simulink model "GCS"  (R2023a)
settings: Solver=ode1  StartTime=0.0  StopTime=inf  FixedStep=1/500  RelTol=1e-3
values from neighbouring files (symbols this model uses):
  data = uint8([                  i_int,                  i_dof,                  typecast(single(t_int), 'uint8'),                  typecast(single(coeffs), 'uint8')])    [trajectory_writer.m]    (also in ulog_plotter.m = topic.sticks(index2plot, i__).Variables)
  res = any(res)    [ulog_parser.m]
undefined symbols (not defined in the file or in its folder): f, FLIGHT_MODE, flight_mode, id, joystick, name, Parameters, timestamp, wait_time_s
libraries: simulink_extras x3, px4uORBlib x2, vrlib x1, uavmavlinklib x1, instrumentlib x1, aerolibanimutils x1
settings Model: Creator=amc0121  LastModifiedBy=yzk0058
settings DebuggingCC: UnconnectedInputMsg=warning  UnconnectedOutputMsg=warning  UnconnectedLineMsg=warning
settings ModelReferenceCC: EnableRefExpFcnMdlSchedulingChecks=on
settings RTWCC: DLArmComputeVersion=19.05

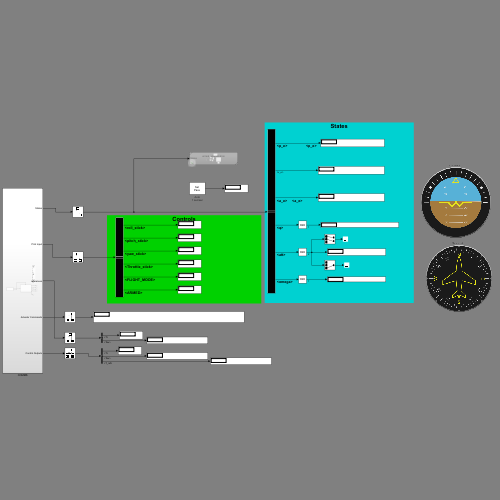
[thumbnail: Simulink's stored preview of the top-level diagram]
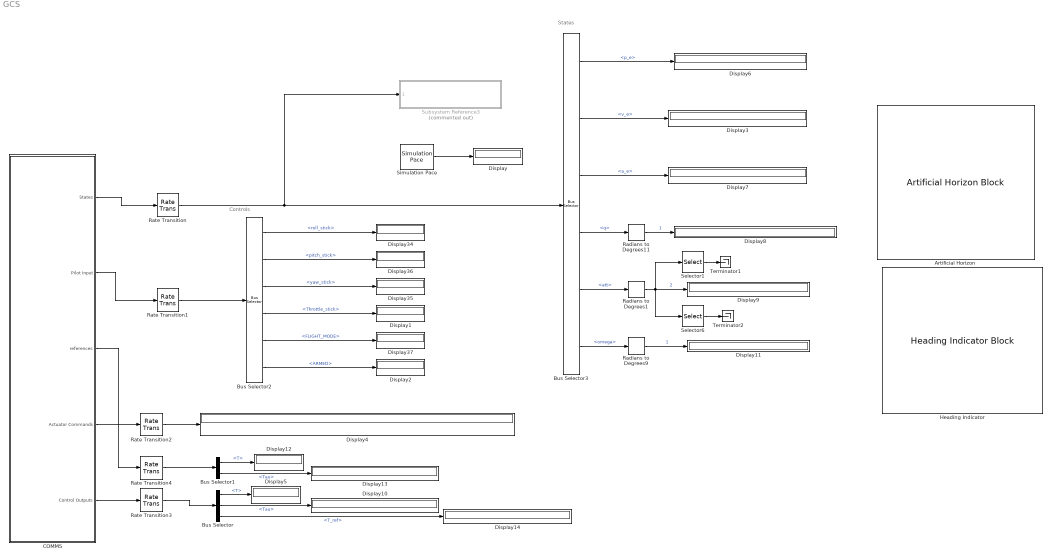
== system GCS ==
  note: Controls
  note: States
  Artificial Horizon : ArtificialHorizonBlock
  Bus Selector : BusSelector  OutputSignals=T,Tau,T_ref
  Bus Selector1 : BusSelector  OutputSignals=reconstructed.T,reconstructed.Tau
  Bus Selector2 : BusSelector  OutputSignals=Pilot Input.Sticks.roll_stick,Pilot Input.Sticks.pitch_stick,Pilot Input.Sticks.yaw_stick,Pilot Input.Sticks.Throttle_stick,Pilot Input.FLIGHT_MODE,Pilot Input.ARMED
  Bus Selector3 : BusSelector  OutputSignals=p_e,v_e,a_e,q,att,omega
  COMMS : Subsystem
  Display{,1..14,34..37} (19 alike) : Display
      Display1 settings: Decimation=30
      Display11 settings: Decimation=30
      Display2 settings: Decimation=30
      Display3 settings: Decimation=30
      Display34 settings: Decimation=30
      Display36 settings: Decimation=30
      Display37 settings: Decimation=30
      Display4 settings: Decimation=30
      Display7 settings: Decimation=30
      Display8 settings: Decimation=30
      Display9 settings: Decimation=30
  Heading Indicator : HeadingIndicatorBlock
  Radians to Degrees1 : simulink_extras/Transformations/Radians to Degrees
  Radians to Degrees11 : simulink_extras/Transformations/Radians to Degrees
  Radians to Degrees9 : simulink_extras/Transformations/Radians to Degrees
  Rate Transition{,1..4} (5 alike) : RateTransition  OutPortSampleTime=1/50
  Selector1 : Selector  InputPortWidth=3  IndexOptions=Index vector (dialog)  Indices=[1 2]  OutputSizes=1
  Selector6 : Selector  InputPortWidth=3  IndexOptions=Index vector (dialog)  Indices=[3]  OutputSizes=1
  Simulation Pace : aerolibanimutils/Simulation Pace  SimulationPace=1  SleepMode=Auto  OutputPaceError=on  SampleTime=-1
  Subsystem Reference3 : Subsystem  Commented=on  ReferencedSubsystem=unreal_visualization
  Terminator1 : Terminator
  Terminator2 : Terminator
  wires:
  Bus Selector3/1 -> Display6/1  "<p_e>"
  Bus Selector3/4 -> Radians to Degrees11/1  "<q>"
  Bus Selector3/3 -> Display7/1  "<a_e>"
  Bus Selector3/5 -> Radians to Degrees1/1  "<att>"
  Bus Selector3/6 -> Radians to Degrees9/1  "<omega>"
  Radians to Degrees9/1 -> Display11/1  "1"
  Radians to Degrees1/1 -> Selector1/1, Selector6/1, Display9/1  "2"
  Radians to Degrees11/1 -> Display8/1  "1"
  Bus Selector2/2 -> Display36/1  "<pitch_stick>"
  Bus Selector2/4 -> Display1/1  "<Throttle_stick>"
  Bus Selector2/6 -> Display2/1  "<ARMED>"
  Bus Selector2/1 -> Display34/1  "<roll_stick>"
  Bus Selector2/3 -> Display35/1  "<yaw_stick>"
  Bus Selector2/5 -> Display37/1  "<FLIGHT_MODE>"
  Simulation Pace/1 -> Display/1
  Selector1/1 -> Terminator1/1
  Selector6/1 -> Terminator2/1
  Bus Selector3/2 -> Display3/1  "<v_e>"
  COMMS/1(States) -> Rate Transition/1
  COMMS/2(Pilot Input) -> Rate Transition1/1
  COMMS/4(Actuator Commands) -> Rate Transition2/1
  Rate Transition2/1 -> Display4/1
  Rate Transition1/1 -> Bus Selector2/1
  Rate Transition/1 -> Subsystem Reference3/1, Bus Selector3/1
  COMMS/5(Control Outputs) -> Rate Transition3/1
  Rate Transition3/1 -> Bus Selector/1
  Bus Selector/1 -> Display5/1  "<T>"
  Bus Selector/2 -> Display10/1  "<Tau>"
  COMMS/3(references) -> Rate Transition4/1
  Rate Transition4/1 -> Bus Selector1/1
  Bus Selector1/1 -> Display12/1  "<T>"
  Bus Selector1/2 -> Display13/1  "<Tau>"
  Bus Selector/3 -> Display14/1  "<T_ref>"

== system GCS/COMMS ==
  note: X Input Order
      | 1. u (Vx)
      | 2. v (Vy)
      | 3. w (Vz)
      | 4. p
      | 5. q
      | 6. r
      | 7. e0
      | 8. e1
      | 9. e2
      | 10. e3
      | 11. Lat
      | 12. Long
      | 13. hMSL
      | 14. hAGL
      | 15. ax
      | 16. ay
      | 17. az
      | 18. x
      | 19. y
      | 20. z
      | 21. hdot (VV)
      | 22. GCFlag
      | 23. TAS
      | 24. EAS
      | 25. LiDAR
  Enabled Subsystem : Subsystem  TreatAsAtomicUnit=on
  UDP Receive : instrumentlib/UDP Receive  LocalAddress=127.0.0.1  LocalPort=14445  EnablePortSharing=off  Host=localhost  Port=9090  GetLatestData=off  DataSize=8  DataType=uint8  ASCIIFormatting=%f,  Terminator=LF  CustomTerminator=10  ByteOrder=big-endian  EnableBlockingMode=off  Timeout=1/300  SampleTime=1/500  SimulateUsing=Interpreted execution
  States : Outport
  Pilot Input : Outport  Port=2
  references : Outport  Port=3
  Actuator Commands : Outport  Port=4
  Control Outputs : Outport  Port=5
  wires:
  UDP Receive/2 -> Enabled Subsystem/Enable
  UDP Receive/1 -> Enabled Subsystem/1(byteStreamInput)
  Enabled Subsystem/1(States) -> States/1
  Enabled Subsystem/2(Pilot Input) -> Pilot Input/1
  Enabled Subsystem/3(references) -> references/1
  Enabled Subsystem/4(Actuator Commands) -> Actuator Commands/1
  Enabled Subsystem/5(Control Outputs) -> Control Outputs/1

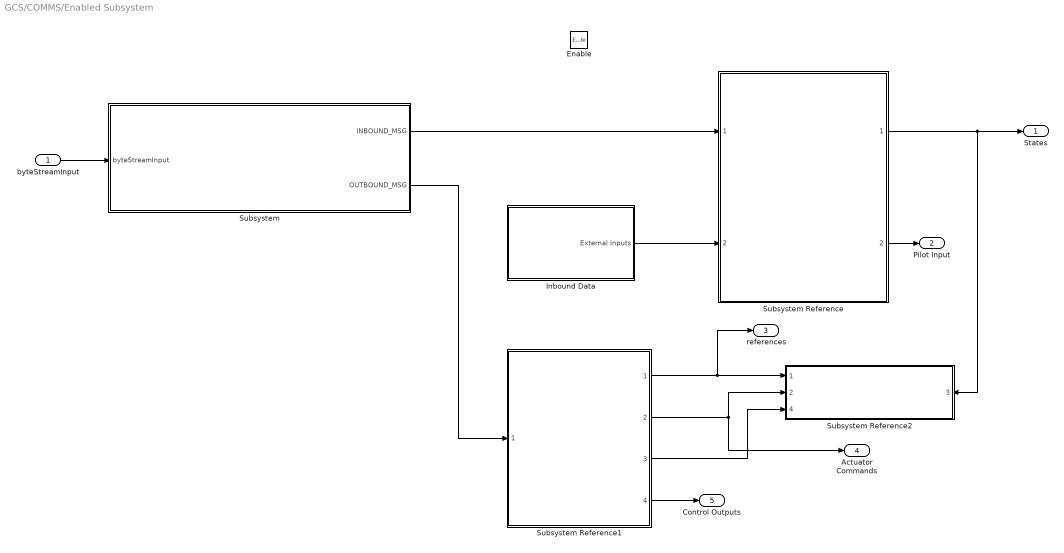
== system GCS/COMMS/Enabled Subsystem ==
  byteStreamInput : Inport
  Enable : EnablePort
  Inbound Data : Subsystem
  Subsystem : Subsystem
  Subsystem Reference : Subsystem  ReferencedSubsystem=INBOUND_MSG_UNMAP
  Subsystem Reference1 : Subsystem  ReferencedSubsystem=OUTBOUND_MSG_UNMAP
  Subsystem Reference2 : Subsystem  ReferencedSubsystem=logging2workspace
      settings: PortSchema="{\"entries\":[{\"content\":{\"sides\":[{\"content\":{\"connectorIds\":[\"In1\",\"In2\",\"In4\"]},\"type\":\"ConnectorPlacement.EquallySpacedRectSide\",\"uuid\":\"47b0435c-4974-4dfb-aae6-6ca620e26367\"},{\"content\":{\"connectorIds\":[\"In3\"],\"side\":\"RIGHT\"},\"type\":\"ConnectorPlacement.EquallySpacedRectSide\",\"uuid\":\"e323305f-4ea2-4fd9-9ec2-838e165181fb\"},{\"content\":{\"side\":\"TOP\"},\"type\":\"ConnectorPlacement.EquallySpacedRectSide\",\"uuid\":\"bec00405-cbc9-4439-89df-ad1a7655b850\"}]},\"type\":\"ConnectorPlacement.EquallySpacedConnector\",\"uuid\":\"1e7e1f21-3d1e-40b5-a907-670aed2a63f6\"}],\"packageUris\":[\"http://schema.mathworks.com/mf0/Connector/R2020b\"],\"version\":\"1.0\"}"
  States : Outport
  Pilot Input : Outport  Port=2
  references : Outport  Port=3
  Actuator Commands : Outport  Port=4
  Control Outputs : Outport  Port=5
  wires:
  byteStreamInput/1 -> Subsystem/1(byteStreamInput)
  Subsystem/2(OUTBOUND_MSG) -> Subsystem Reference1/1
  Subsystem/1(INBOUND_MSG) -> Subsystem Reference/1
  Inbound Data/1("External Inputs ") -> Subsystem Reference/2
  Subsystem Reference/1 -> States/1, Subsystem Reference2/3
  Subsystem Reference1/1 -> references/1, Subsystem Reference2/1
  Subsystem Reference/2 -> Pilot Input/1
  Subsystem Reference1/2 -> Actuator Commands/1, Subsystem Reference2/2
  Subsystem Reference1/3 -> Subsystem Reference2/4
  Subsystem Reference1/4 -> Control Outputs/1

== system GCS/COMMS/Enabled Subsystem/Inbound Data ==
  Bus Creator3 : BusCreator  Inputs=4
  Subsystem1 : Subsystem
  Subsystem2 : Subsystem
  Subsystem3 : Subsystem
  Subsystem4 : Subsystem
  "External Inputs " : Outport
  wires:
  Bus Creator3/1 -> "External Inputs "/1
  Subsystem1/1(Control Gains) -> Bus Creator3/2  "Control Gains"
  Subsystem2/1(Vehicle Parameters) -> Bus Creator3/1  "Vehicle Parameters"
  Subsystem3/1(Trajectory) -> Bus Creator3/3  "Trajectory"
  Subsystem4/1(Pilot Input) -> Bus Creator3/4  "Pilot Input"

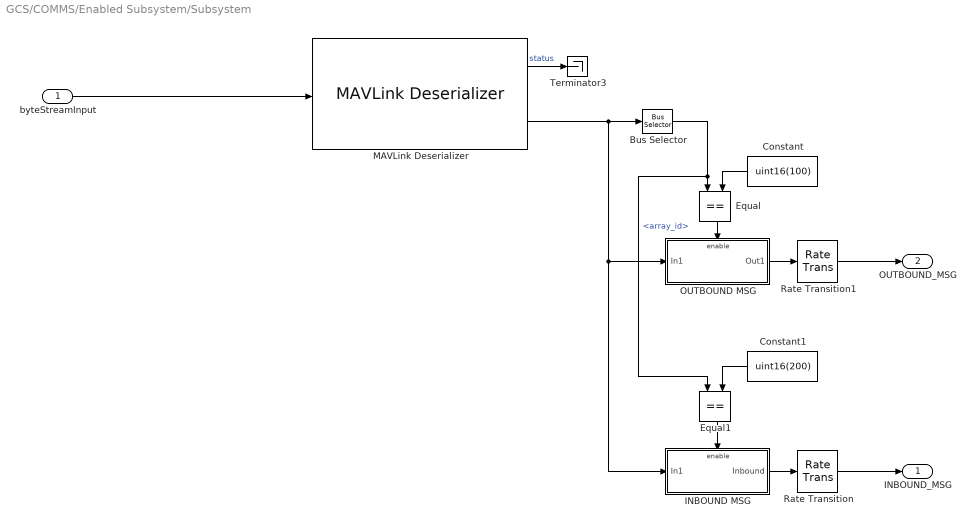
== system GCS/COMMS/Enabled Subsystem/Subsystem ==
  byteStreamInput : Inport
  Bus Selector : BusSelector  OutputSignals=Payload.array_id
  Constant : Constant  Value=uint16(100)
  Constant1 : Constant  Value=uint16(200)
  Equal : RelationalOperator  Operator===  OutDataTypeStr=boolean  RndMeth=Simplest  InputSameDT=off
  Equal1 : RelationalOperator  Operator===  OutDataTypeStr=boolean  RndMeth=Simplest  InputSameDT=off
  INBOUND MSG : Subsystem  TreatAsAtomicUnit=on
  MAVLink Deserializer : uavmavlinklib/MAVLink Deserializer  dialectSource=Select from standard MAVLink dialects  dialect=common.xml  dialectCustom=common.xml  version=2  messageType=DEBUG_FLOAT_ARRAY  inputDataLength=off  SystemIDFilter=off  systemID=1  ComponentIDFilter=off  componentID=1  queueMsg=off  queueMsgSize=50  dropNum=off
  OUTBOUND MSG : Subsystem  TreatAsAtomicUnit=on
  Rate Transition : RateTransition  OutPortSampleTime=1/25
  Rate Transition1 : RateTransition  OutPortSampleTime=1/25
  Terminator3 : Terminator
  INBOUND_MSG : Outport
  OUTBOUND_MSG : Outport  Port=2
  wires:
  Equal1/1 -> INBOUND MSG/Enable
  INBOUND MSG/1(Inbound) -> Rate Transition/1
  OUTBOUND MSG/1(Out1) -> Rate Transition1/1
  MAVLink Deserializer/2 -> INBOUND MSG/1(In1), OUTBOUND MSG/1(In1), Bus Selector/1
  Bus Selector/1 -> Equal1/1, Equal/1  "<array_id>"
  Constant/1 -> Equal/2
  Equal/1 -> OUTBOUND MSG/Enable
  Rate Transition/1 -> INBOUND_MSG/1
  MAVLink Deserializer/1 -> Terminator3/1  "status"
  Constant1/1 -> Equal1/2
  byteStreamInput/1 -> MAVLink Deserializer/1
  Rate Transition1/1 -> OUTBOUND_MSG/1

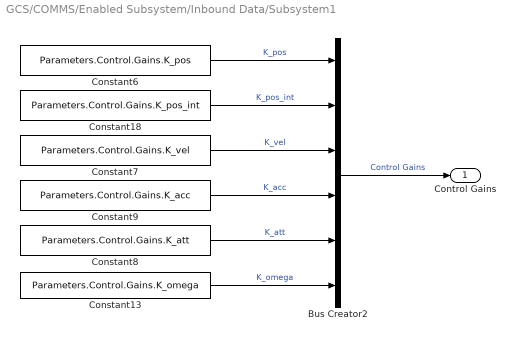
== system GCS/COMMS/Enabled Subsystem/Inbound Data/Subsystem1 ==
  Bus Creator2 : BusCreator  Inputs=6
  Constant13 : Constant  Value=Parameters.Control.Gains.K_omega
  Constant18 : Constant  Value=Parameters.Control.Gains.K_pos_int
  Constant6 : Constant  Value=Parameters.Control.Gains.K_pos
  Constant7 : Constant  Value=Parameters.Control.Gains.K_vel
  Constant8 : Constant  Value=Parameters.Control.Gains.K_att
  Constant9 : Constant  Value=Parameters.Control.Gains.K_acc
  Control Gains : Outport
  wires:
  Constant7/1 -> Bus Creator2/3  "K_vel"
  Constant6/1 -> Bus Creator2/1  "K_pos"
  Constant13/1 -> Bus Creator2/6  "K_omega"
  Bus Creator2/1 -> Control Gains/1  "Control Gains"
  Constant18/1 -> Bus Creator2/2  "K_pos_int"
  Constant9/1 -> Bus Creator2/4  "K_acc"
  Constant8/1 -> Bus Creator2/5  "K_att"

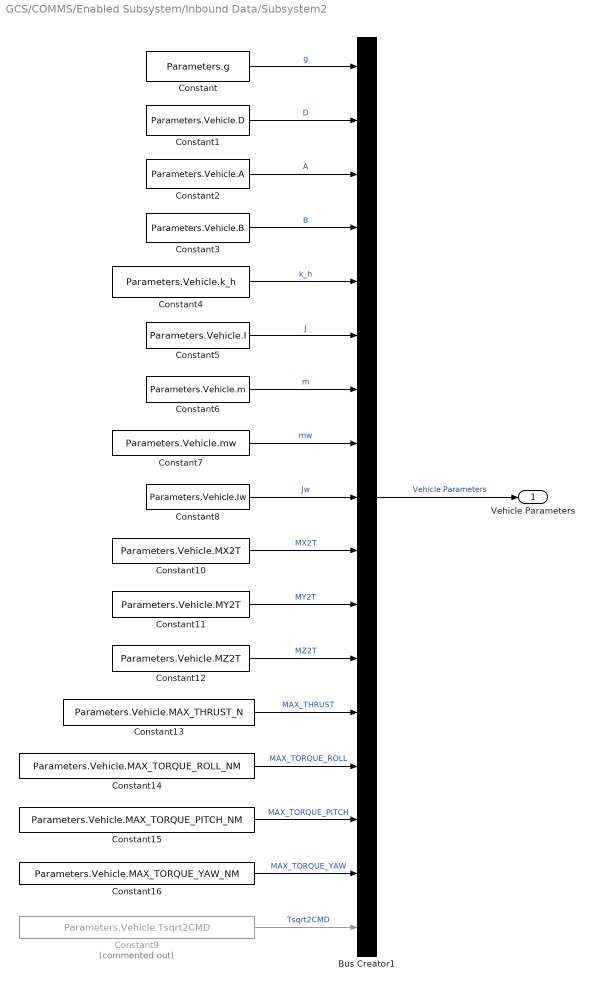
== system GCS/COMMS/Enabled Subsystem/Inbound Data/Subsystem2 ==
  Bus Creator1 : BusCreator  Inputs=17
  Constant : Constant  Value=Parameters.g
  Constant1 : Constant  Value=Parameters.Vehicle.D
  Constant10 : Constant  Value=Parameters.Vehicle.MX2T
  Constant11 : Constant  Value=Parameters.Vehicle.MY2T
  Constant12 : Constant  Value=Parameters.Vehicle.MZ2T
  Constant13 : Constant  Value=Parameters.Vehicle.MAX_THRUST_N
  Constant14 : Constant  Value=Parameters.Vehicle.MAX_TORQUE_ROLL_NM
  Constant15 : Constant  Value=Parameters.Vehicle.MAX_TORQUE_PITCH_NM
  Constant16 : Constant  Value=Parameters.Vehicle.MAX_TORQUE_YAW_NM
  Constant2 : Constant  Value=Parameters.Vehicle.A
  Constant3 : Constant  Value=Parameters.Vehicle.B
  Constant4 : Constant  Value=Parameters.Vehicle.k_h
  Constant5 : Constant  Value=Parameters.Vehicle.I
  Constant6 : Constant  Value=Parameters.Vehicle.m
  Constant7 : Constant  Value=Parameters.Vehicle.mw
  Constant8 : Constant  Value=Parameters.Vehicle.Iw
  Constant9 : Constant  Commented=on  Value=Parameters.Vehicle.Tsqrt2CMD
  Vehicle Parameters : Outport
  wires:
  Constant5/1 -> Bus Creator1/6  "J"
  Constant3/1 -> Bus Creator1/4  "B"
  Constant/1 -> Bus Creator1/1  "g"
  Constant1/1 -> Bus Creator1/2  "D"
  Constant2/1 -> Bus Creator1/3  "A"
  Constant4/1 -> Bus Creator1/5  "k_h"
  Bus Creator1/1 -> Vehicle Parameters/1  "Vehicle Parameters"
  Constant6/1 -> Bus Creator1/7  "m"
  Constant7/1 -> Bus Creator1/8  "mw"
  Constant8/1 -> Bus Creator1/9  "Jw"
  Constant10/1 -> Bus Creator1/10  "MX2T"
  Constant11/1 -> Bus Creator1/11  "MY2T"
  Constant12/1 -> Bus Creator1/12  "MZ2T"
  Constant13/1 -> Bus Creator1/13  "MAX_THRUST"
  Constant14/1 -> Bus Creator1/14  "MAX_TORQUE_ROLL"
  Constant15/1 -> Bus Creator1/15  "MAX_TORQUE_PITCH"
  Constant16/1 -> Bus Creator1/16  "MAX_TORQUE_YAW"
  Constant9/1 -> Bus Creator1/17  "Tsqrt2CMD"

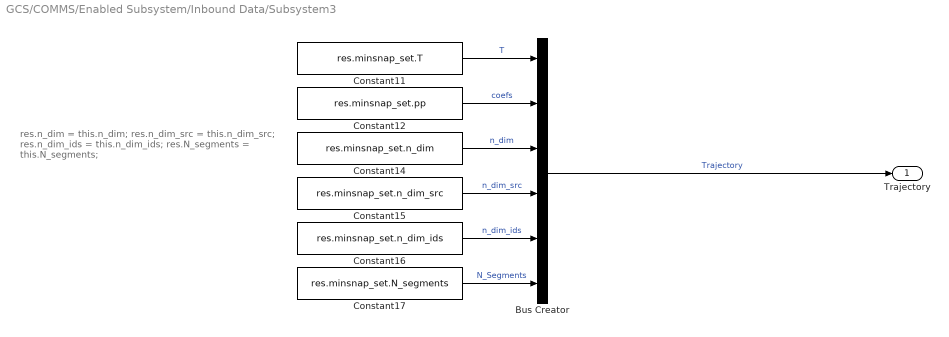
== system GCS/COMMS/Enabled Subsystem/Inbound Data/Subsystem3 ==
  note: res.n_dim = this.n_dim;
      | res.n_dim_src = this.n_dim_src;
      | res.n_dim_ids = this.n_dim_ids;
      | res.N_segments = this.N_segments;
  Bus Creator : BusCreator  Inputs=6
  Constant11 : Constant  Value=res.minsnap_set.T
  Constant12 : Constant  Value=res.minsnap_set.pp
  Constant14 : Constant  Value=res.minsnap_set.n_dim
  Constant15 : Constant  Value=res.minsnap_set.n_dim_src
  Constant16 : Constant  Value=res.minsnap_set.n_dim_ids
  Constant17 : Constant  Value=res.minsnap_set.N_segments
  Trajectory : Outport
  wires:
  Constant12/1 -> Bus Creator/2  "coefs"
  Constant14/1 -> Bus Creator/3  "n_dim"
  Constant11/1 -> Bus Creator/1  "T"
  Constant16/1 -> Bus Creator/5  "n_dim_ids"
  Bus Creator/1 -> Trajectory/1  "Trajectory"
  Constant15/1 -> Bus Creator/4  "n_dim_src"
  Constant17/1 -> Bus Creator/6  "N_Segments"

== system GCS/COMMS/Enabled Subsystem/Inbound Data/Subsystem4 ==
  Bus Creator4 : BusCreator  Inputs=4
  Subsystem : Subsystem
  Subsystem1 : Subsystem
  Pilot Input : Outport
  wires:
  Subsystem/1(sticks) -> Bus Creator4/1  "Sticks"
  Bus Creator4/1 -> Pilot Input/1  "Pilot Input"
  Subsystem1/1(Parameters) -> Bus Creator4/4  "Parameters"
  Subsystem/2(FLIGHT_MODE) -> Bus Creator4/2  "FLIGHT_MODE"
  Subsystem/3(ARMED) -> Bus Creator4/3  "ARMED"

== system GCS/COMMS/Enabled Subsystem/Subsystem/INBOUND MSG ==
  In1 : Inport
  Enable : EnablePort
  Bus Assignment : BusAssignment  AssignedSignals=timestamp,data,id,name
  Bus Selector1 : BusSelector  OutputSignals=Payload.time_usec,Payload.data,Payload.array_id,Payload.name
  PX4 uORB Message : px4uORBlib/PX4 uORB Message  uORBTopic=debug_array  SampleTime=inf  selectInstance=vehicle_gps_position
  Inbound : Outport
  wires:
  Bus Selector1/4 -> Bus Assignment/5  "<name>"
  Bus Selector1/3 -> Bus Assignment/4  "<array_id>"
  Bus Assignment/1 -> Inbound/1
  Bus Selector1/1 -> Bus Assignment/2  "<time_usec>"
  Bus Selector1/2 -> Bus Assignment/3  "<data>"
  In1/1 -> Bus Selector1/1
  PX4 uORB Message/1 -> Bus Assignment/1

== system GCS/COMMS/Enabled Subsystem/Subsystem/OUTBOUND MSG ==
  In1 : Inport
  Enable : EnablePort
  Bus Assignment : BusAssignment  AssignedSignals=timestamp,data,id,name
  Bus Selector1 : BusSelector  OutputSignals=Payload.time_usec,Payload.data,Payload.array_id,Payload.name
  PX4 uORB Message : px4uORBlib/PX4 uORB Message  uORBTopic=debug_array  SampleTime=inf  selectInstance=vehicle_gps_position
  Out1 : Outport
  wires:
  Bus Selector1/2 -> Bus Assignment/3  "<data>"
  Bus Selector1/1 -> Bus Assignment/2  "<time_usec>"
  Bus Selector1/3 -> Bus Assignment/4  "<array_id>"
  PX4 uORB Message/1 -> Bus Assignment/1
  In1/1 -> Bus Selector1/1
  Bus Selector1/4 -> Bus Assignment/5  "<name>"
  Bus Assignment/1 -> Out1/1

== system GCS/COMMS/Enabled Subsystem/Inbound Data/Subsystem4/Subsystem ==
  Bus Creator4 : BusCreator  Inputs=4
  Subsystem1 : Subsystem  Variant=on  VariantControlMode=label  VariantControl=Choice  LabelModeActiveChoice=Choice_1
  sticks : Outport
  FLIGHT_MODE : Outport  Port=2
  ARMED : Outport  Port=3
  wires:
  Bus Creator4/1 -> sticks/1
  Subsystem1/1(roll_stick) -> Bus Creator4/1
  Subsystem1/2(pitch_stick) -> Bus Creator4/2
  Subsystem1/3(yaw_stick) -> Bus Creator4/3
  Subsystem1/4(Throttle_stick) -> Bus Creator4/4
  Subsystem1/5(FLIGHT_MODE) -> FLIGHT_MODE/1
  Subsystem1/6(ARMED) -> ARMED/1

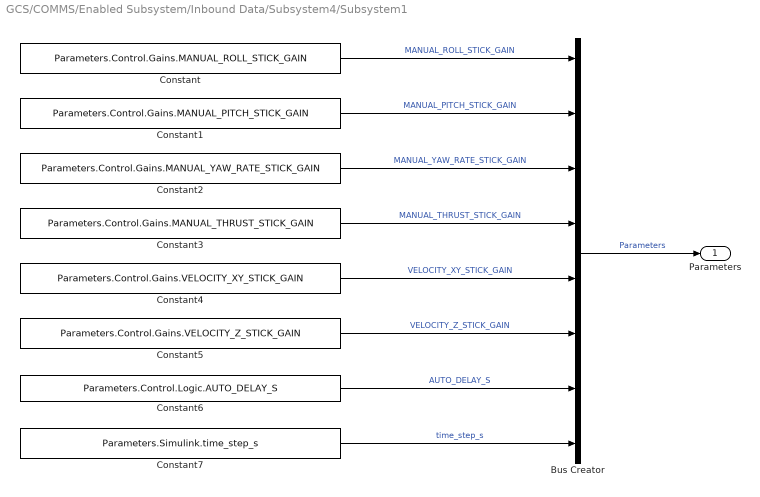
== system GCS/COMMS/Enabled Subsystem/Inbound Data/Subsystem4/Subsystem1 ==
  Bus Creator : BusCreator  Inputs=8
  Constant : Constant  Value=Parameters.Control.Gains.MANUAL_ROLL_STICK_GAIN
  Constant1 : Constant  Value=Parameters.Control.Gains.MANUAL_PITCH_STICK_GAIN
  Constant2 : Constant  Value=Parameters.Control.Gains.MANUAL_YAW_RATE_STICK_GAIN
  Constant3 : Constant  Value=Parameters.Control.Gains.MANUAL_THRUST_STICK_GAIN
  Constant4 : Constant  Value=Parameters.Control.Gains.VELOCITY_XY_STICK_GAIN
  Constant5 : Constant  Value=Parameters.Control.Gains.VELOCITY_Z_STICK_GAIN
  Constant6 : Constant  Value=Parameters.Control.Logic.AUTO_DELAY_S
  Constant7 : Constant  Value=Parameters.Simulink.time_step_s
  Parameters : Outport
  wires:
  Constant/1 -> Bus Creator/1  "MANUAL_ROLL_STICK_GAIN"
  Bus Creator/1 -> Parameters/1  "Parameters"
  Constant1/1 -> Bus Creator/2  "MANUAL_PITCH_STICK_GAIN"
  Constant2/1 -> Bus Creator/3  "MANUAL_YAW_RATE_STICK_GAIN"
  Constant3/1 -> Bus Creator/4  "MANUAL_THRUST_STICK_GAIN"
  Constant4/1 -> Bus Creator/5  "VELOCITY_XY_STICK_GAIN"
  Constant5/1 -> Bus Creator/6  "VELOCITY_Z_STICK_GAIN"
  Constant6/1 -> Bus Creator/7  "AUTO_DELAY_S"
  Constant7/1 -> Bus Creator/8  "time_step_s"

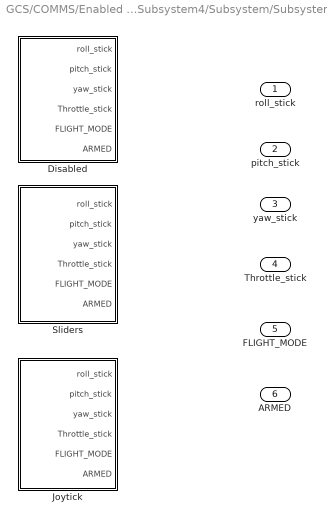
== system GCS/COMMS/Enabled Subsystem/Inbound Data/Subsystem4/Subsystem/Subsystem1 ==
  Disabled : Subsystem  VariantControl=Choice_1
  Joytick : Subsystem  VariantControl=Choice
  Sliders : Subsystem  VariantControl=Choice_2
  roll_stick : Outport
  pitch_stick : Outport  Port=2
  yaw_stick : Outport  Port=3
  Throttle_stick : Outport  Port=4
  FLIGHT_MODE : Outport  Port=5
  ARMED : Outport  Port=6

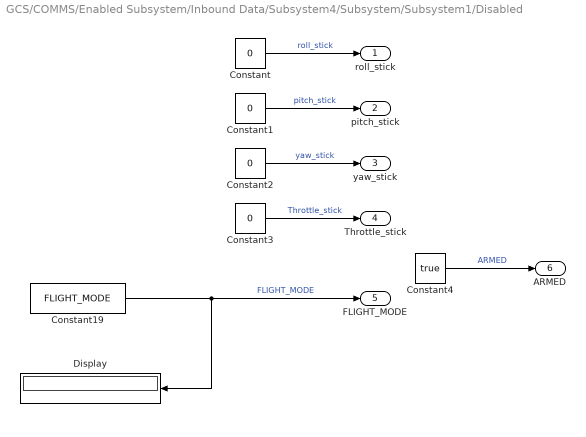
== system GCS/COMMS/Enabled Subsystem/Inbound Data/Subsystem4/Subsystem/Subsystem1/Disabled ==
  Constant{,1..3} (4 alike) : Constant  Value=0
  Constant19 : Constant  Value=FLIGHT_MODE
  Constant4 : Constant  Value=true
  Display : Display
  roll_stick : Outport
  pitch_stick : Outport  Port=2
  yaw_stick : Outport  Port=3
  Throttle_stick : Outport  Port=4
  FLIGHT_MODE : Outport  Port=5
  ARMED : Outport  Port=6
  wires:
  Constant3/1 -> Throttle_stick/1  "Throttle_stick"
  Constant1/1 -> pitch_stick/1  "pitch_stick"
  Constant/1 -> roll_stick/1  "roll_stick"
  Constant2/1 -> yaw_stick/1  "yaw_stick"
  Constant19/1 -> FLIGHT_MODE/1, Display/1  "FLIGHT_MODE"
  Constant4/1 -> ARMED/1  "ARMED"

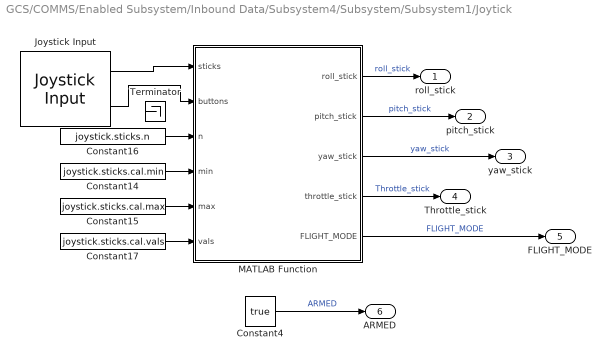
== system GCS/COMMS/Enabled Subsystem/Inbound Data/Subsystem4/Subsystem/Subsystem1/Joytick ==
  Constant14 : Constant  Value=joystick.sticks.cal.min
  Constant15 : Constant  Value=joystick.sticks.cal.max
  Constant16 : Constant  Value=joystick.sticks.n
  Constant17 : Constant  Value=joystick.sticks.cal.vals
  Constant4 : Constant  Value=true
  Joystick Input : vrlib/Joystick Input  joyid=1  adjustports=on  forcefeed=off
  MATLAB Function : MATLAB Function  TreatAsAtomicUnit=on
  Terminator : Terminator
  roll_stick : Outport
  pitch_stick : Outport  Port=2
  yaw_stick : Outport  Port=3
  Throttle_stick : Outport  Port=4
  FLIGHT_MODE : Outport  Port=5
  ARMED : Outport  Port=6
  wires:
  Constant15/1 -> MATLAB Function/5(max)
  Constant14/1 -> MATLAB Function/4(min)
  MATLAB Function/4(throttle_stick) -> Throttle_stick/1  "Throttle_stick"
  Constant16/1 -> MATLAB Function/3(n)
  Constant17/1 -> MATLAB Function/6(vals)
  Joystick Input/1 -> MATLAB Function/1(sticks)
  MATLAB Function/2(pitch_stick) -> pitch_stick/1  "pitch_stick"
  Joystick Input/2 -> MATLAB Function/2(buttons)
  ? -> Terminator/1
  MATLAB Function/1(roll_stick) -> roll_stick/1  "roll_stick"
  MATLAB Function/3(yaw_stick) -> yaw_stick/1  "yaw_stick"
  MATLAB Function/5(FLIGHT_MODE) -> FLIGHT_MODE/1  "FLIGHT_MODE"
  Constant4/1 -> ARMED/1  "ARMED"

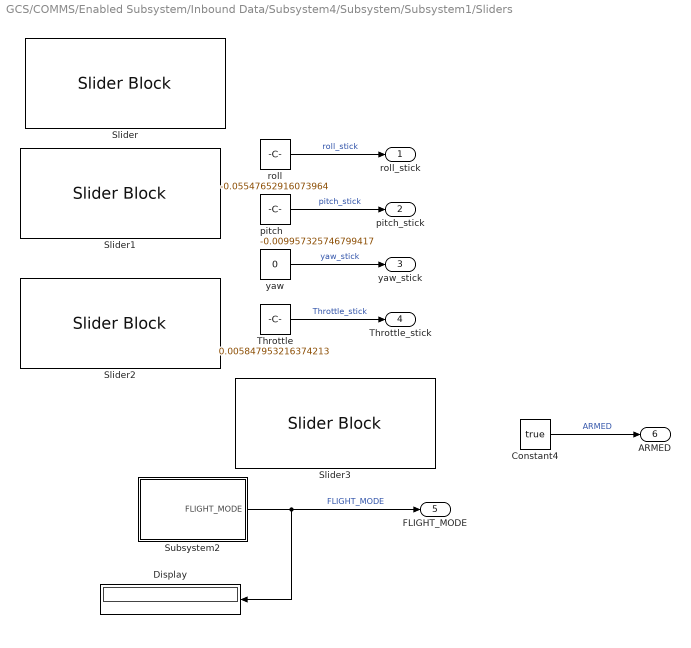
== system GCS/COMMS/Enabled Subsystem/Inbound Data/Subsystem4/Subsystem/Subsystem1/Sliders ==
  Constant4 : Constant  Value=true
  Display : Display
  Slider{,1..3} (4 alike) : SliderBlock  ScaleMin=-1  ScaleMax=1
  Subsystem2 : Subsystem
  Throttle : Constant  Value=0.005847953216374213
  pitch : Constant  Value=-0.009957325746799417
  roll : Constant  Value=-0.05547652916073964
  yaw : Constant  Value=0
  roll_stick : Outport
  pitch_stick : Outport  Port=2
  yaw_stick : Outport  Port=3
  Throttle_stick : Outport  Port=4
  FLIGHT_MODE : Outport  Port=5
  ARMED : Outport  Port=6
  wires:
  roll/1 -> roll_stick/1  "roll_stick"
  yaw/1 -> yaw_stick/1  "yaw_stick"
  pitch/1 -> pitch_stick/1  "pitch_stick"
  Throttle/1 -> Throttle_stick/1  "Throttle_stick"
  Subsystem2/1(FLIGHT_MODE) -> FLIGHT_MODE/1, Display/1  "FLIGHT_MODE"
  Constant4/1 -> ARMED/1  "ARMED"

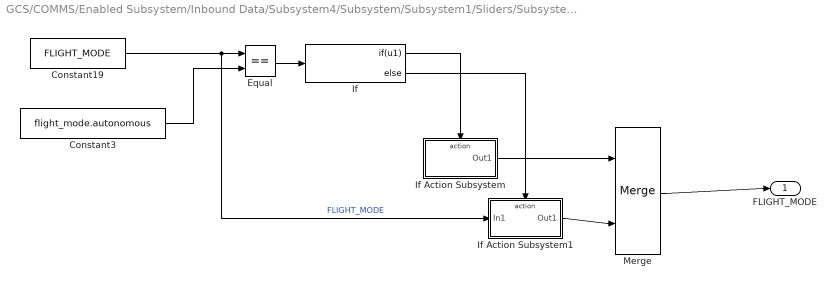
== system GCS/COMMS/Enabled Subsystem/Inbound Data/Subsystem4/Subsystem/Subsystem1/Sliders/Subsystem2 ==
  Constant19 : Constant  Value=FLIGHT_MODE
  Constant3 : Constant  Value=flight_mode.autonomous
  Equal : RelationalOperator  Operator===  OutDataTypeStr=boolean  RndMeth=Simplest  InputSameDT=off
  If : If  IfExpression=u1
  If Action Subsystem : Subsystem  TreatAsAtomicUnit=on
  If Action Subsystem1 : Subsystem  TreatAsAtomicUnit=on
  Merge : Merge
  FLIGHT_MODE : Outport
  wires:
  If/1 -> If Action Subsystem/Action
  If Action Subsystem1/1(Out1) -> Merge/2
  Merge/1 -> FLIGHT_MODE/1
  Constant19/1 -> If Action Subsystem1/1(In1), Equal/1  "FLIGHT_MODE"
  Constant3/1 -> Equal/2
  Equal/1 -> If/1
  If/2 -> If Action Subsystem1/Action
  If Action Subsystem/1(Out1) -> Merge/1

== system GCS/COMMS/Enabled Subsystem/Inbound Data/Subsystem4/Subsystem/Subsystem1/Sliders/Subsystem2/If Action Subsystem ==
  Action Port : ActionPort
  Clock : Clock
  Constant : Constant  Value=flight_mode.autonomous
  Constant1 : Constant  Value=flight_mode.position_hold
  Constant2 : Constant  Value=wait_time_s
  GreaterThan : RelationalOperator  Operator=<  OutDataTypeStr=boolean  RndMeth=Simplest  InputSameDT=off
  Multiport Switch1 : MultiPortSwitch  DataPortOrder=Zero-based contiguous  Inputs=2  DiagnosticForDefault=None  zeroidx=on  SaturateOnIntegerOverflow=off  InputSameDT=off
  Out1 : Outport
  wires:
  Constant2/1 -> GreaterThan/2
  Constant1/1 -> Multiport Switch1/3
  GreaterThan/1 -> Multiport Switch1/1
  Constant/1 -> Multiport Switch1/2
  Multiport Switch1/1 -> Out1/1
  Clock/1 -> GreaterThan/1

== system GCS/COMMS/Enabled Subsystem/Inbound Data/Subsystem4/Subsystem/Subsystem1/Sliders/Subsystem2/If Action Subsystem1 ==
  In1 : Inport
  Action Port : ActionPort
  Out1 : Outport
  wires:
  In1/1 -> Out1/1

== matlab function GCS/COMMS/Enabled Subsystem/Inbound Data/Subsystem4/Subsystem/Subsystem1/Joytick/MATLAB Function ==
  data: sticks input; roll_stick output; buttons input; n input; min input; max input; pitch_stick output; yaw_stick output; throttle_stick output; vals input; FLIGHT_MODE output
function [roll_stick, pitch_stick, yaw_stick, throttle_stick, FLIGHT_MODE] = fcn(sticks, buttons, n, min, max, vals)
joystick.sticks.raw = sticks;
joystick.buttons.raw = buttons;
joystick.sticks.n = n;
joystick.sticks.cal.min = min;
joystick.sticks.cal.max = max;
joystick.sticks.cal.vals = vals;

ROLL_STICK = 1;
PITCH_STICK = 2;
THROTTLE_STICK = 3;
YAW_STICK = 5;
AUX1_STICK = 4;

StickMap = [...
    ROLL_STICK
    PITCH_STICK
    YAW_STICK
    THROTTLE_STICK
    AUX1_STICK];

ROLL_STICK_POL = 1;
PITCH_STICK_POL = -1;
THROTTLE_STICK_POL = -1;
YAW_STICK_POL = 1;
AUX1_STICK_POL = 1;

StickPol = [...
    ROLL_STICK_POL
    PITCH_STICK_POL
    YAW_STICK_POL
    THROTTLE_STICK_POL
    AUX1_STICK_POL];

% tol = 1E-12;
deadzone_RPY = 0.05; %sticks are not perfectly centered 
deadzone_Z = 0.05;
joystick = lib.joystick.apply_cal(joystick);
mapped_sticks = joystick.sticks.cal.vals(StickMap);
mapped_sticks = mapped_sticks(:).*StickPol(:);
roll_stick = lib.math.apply_deadzone(mapped_sticks(1),deadzone_RPY,0);
pitch_stick = lib.math.apply_deadzone(mapped_sticks(2),deadzone_RPY,0);
yaw_stick = lib.math.apply_deadzone(mapped_sticks(3),deadzone_RPY,0);
throttle_stick = lib.math.apply_deadzone(mapped_sticks(4),deadzone_Z,0);

button_case = 0;
flight_mode_buttons = buttons(4:5);
if flight_mode_buttons(1) == 0 && flight_mode_buttons(2) == 0
    button_case = 0;
elseif flight_mode_buttons(1) == 1
    button_case = 1;
elseif flight_mode_buttons(2) == 1
    button_case = 2;
end


switch button_case
    case 2
        FLIGHT_MODE = flight_mode.autonomous;
    case 1
        FLIGHT_MODE = flight_mode.attitude_control;
        % FLIGHT_MODE = flight_mode.position_control;
    case 0
        % FLIGHT_MODE = flight_mode.attitude_control;
        FLIGHT_MODE = flight_mode.position_control;
    otherwise 
        FLIGHT_MODE = flight_mode.position_hold;
end

end
